simulink model "cav_pid"  (R2026b)
settings: Solver=ode4  StopTime=P.Tsim  FixedStep=P.dt
InitFcn:
  | P = cav_params(); road = make_road(P.road.segments, P.road.ds, P.road.transition); mpcverbosity off;
libraries: slpidlib x3, autolibshared x1
settings Model: Creator=za  LastModifiedBy=za
settings SolverCC: AutoInsertRateTranBlk=on

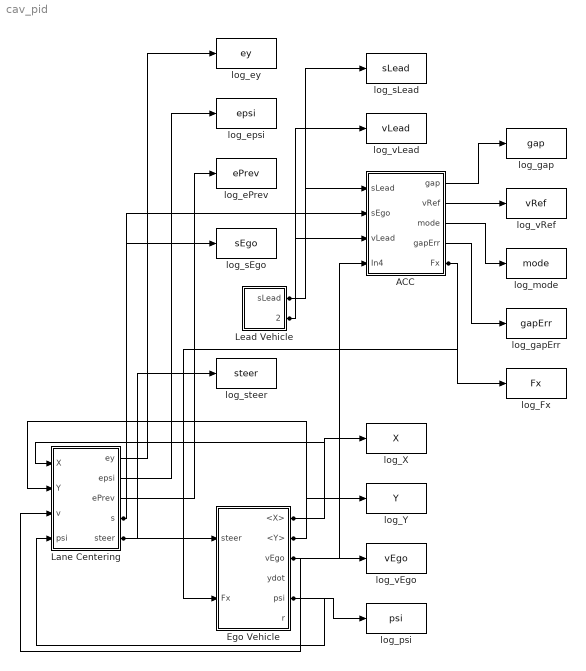
== system cav_pid ==
  ACC : Subsystem
  Ego Vehicle : Subsystem
  Lane Centering : Subsystem
  Lead Vehicle : Subsystem
  log_Fx : ToWorkspace  VariableName=Fx  SaveFormat=Timeseries  SampleTime=P.Ts
  log_X : ToWorkspace  VariableName=X  SaveFormat=Timeseries  SampleTime=P.Ts
  log_Y : ToWorkspace  VariableName=Y  SaveFormat=Timeseries  SampleTime=P.Ts
  log_ePrev : ToWorkspace  VariableName=ePrev  SaveFormat=Timeseries  SampleTime=P.Ts
  log_epsi : ToWorkspace  VariableName=epsi  SaveFormat=Timeseries  SampleTime=P.Ts
  log_ey : ToWorkspace  VariableName=ey  SaveFormat=Timeseries  SampleTime=P.Ts
  log_gap : ToWorkspace  VariableName=gap  SaveFormat=Timeseries  SampleTime=P.Ts
  log_gapErr : ToWorkspace  VariableName=gapErr  SaveFormat=Timeseries  SampleTime=P.Ts
  log_mode : ToWorkspace  VariableName=mode  SaveFormat=Timeseries  SampleTime=P.Ts
  log_psi : ToWorkspace  VariableName=psi  SaveFormat=Timeseries  SampleTime=P.Ts
  log_sEgo : ToWorkspace  VariableName=sEgo  SaveFormat=Timeseries  SampleTime=P.Ts
  log_sLead : ToWorkspace  VariableName=sLead  SaveFormat=Timeseries  SampleTime=P.Ts
  log_steer : ToWorkspace  VariableName=steer  SaveFormat=Timeseries  SampleTime=P.Ts
  log_vEgo : ToWorkspace  VariableName=vEgo  SaveFormat=Timeseries  SampleTime=P.Ts
  log_vLead : ToWorkspace  VariableName=vLead  SaveFormat=Timeseries  SampleTime=P.Ts
  log_vRef : ToWorkspace  VariableName=vRef  SaveFormat=Timeseries  SampleTime=P.Ts
  wires:
  ACC/4(gapErr) -> log_gapErr/1
  ACC/3(mode) -> log_mode/1
  ACC/5(Fx) -> log_Fx/1, Ego Vehicle/2(Fx)
  Lane Centering/5(steer) -> Ego Vehicle/1(steer), log_steer/1
  Lane Centering/1(ey) -> log_ey/1
  Lane Centering/2(epsi) -> log_epsi/1
  Ego Vehicle/2(<Y>) -> log_Y/1, Lane Centering/2(Y)
  Lane Centering/3(ePrev) -> log_ePrev/1
  Lead Vehicle/2(vLead) -> log_vLead/1, ACC/3(vLead)
  ACC/2(vRef) -> log_vRef/1
  Lane Centering/4(s) -> log_sEgo/1, ACC/2(sEgo)
  Lead Vehicle/1(sLead) -> ACC/1(sLead), log_sLead/1
  Ego Vehicle/5(psi) -> log_psi/1, Lane Centering/4(psi)
  Ego Vehicle/3(vEgo) -> log_vEgo/1, ACC/4(In4), Lane Centering/3(v)
  Ego Vehicle/1(<X>) -> log_X/1, Lane Centering/1(X)
  ACC/1(gap) -> log_gap/1

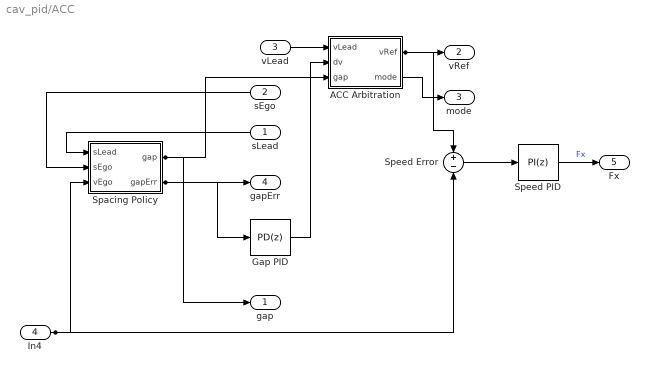
== system cav_pid/ACC ==
  sLead : Inport
  sEgo : Inport  Port=2
  vLead : Inport  Port=3
  In4 : Inport  Port=4
  ACC Arbitration : MATLAB Function  TreatAsAtomicUnit=on
  Gap PID : slpidlib/PID Controller  Controller=PD  Form=Parallel  TimeDomain=Discrete-time  UseExternalTs=off  SampleTime=P.Ts  IntegratorMethod=Forward Euler  FilterMethod=Backward Euler  ControllerParametersSource=internal  P=P.acc.gap.P  I=1  UseKiTs=off  D=P.acc.gap.D  UseExternalDerivativeSource=off  N=P.acc.gap.N  UseFilter=on  TunerSelectOption=Transfer Function Based (PID Tuner App)  InitialConditionSource=internal  InitialConditionForIntegrator=0  InitialConditionForFilter=0  DifferentiatorICPrevScaledInput=0  ExternalReset=none  TrackingMode=off  Kt=1  LimitOutput=on  SatLimitsSource=internal  UpperSaturationLimit=P.acc.gap.dvMax  LowerSaturationLimit=-P.acc.gap.dvMax  LinearizeAsGain=off  AntiWindupMode=none  Kb=1  LimitIntegrator=off  UpperIntegratorSaturationLimit=inf  LowerIntegratorSaturationLimit=-inf  POutMin=[]  POutMax=[]  IOutMin=[]  IOutMax=[]  DOutMin=[]  DOutMax=[]  NOutMin=[]  NOutMax=[]  SumOutMin=[]  SumOutMax=[]  SaturationOutMin=[]  SaturationOutMax=[]  PParamMin=[]  PParamMax=[]  IParamMin=[]  IParamMax=[]  DParamMin=[]  DParamMax=[]  NParamMin=[]  NParamMax=[]  KbParamMin=[]  KbParamMax=[]  KtParamMin=[]  KtParamMax=[]  KbOutMin=[]  KbOutMax=[]  KtOutMin=[]  KtOutMax=[]  IntegratorOutMin=[]  IntegratorOutMax=[]  FilterOutMin=[]  FilterOutMax=[]  SumI1OutMin=[]  SumI1OutMax=[]  SumI2OutMin=[]  SumI2OutMax=[]  SumI3OutMin=[]  SumI3OutMax=[]  SumI4OutMin=[]  SumI4OutMax=[]  SumDOutMin=[]  SumDOutMax=[]  DifferentiatorOutMin=[]  DifferentiatorOutMax=[]  FilterDiffOutCoefMin=[]  FilterDiffOutCoefMax=[]  ReciprocalOutMin=[]  ReciprocalOutMax=[]  SumDenOutMin=[]  SumDenOutMax=[]  SumNumOutMin=[]  SumNumOutMax=[]  DivideOutMin=[]  DivideOutMax=[]  UdiffTsProdOutMin=[]  UdiffTsProdOutMax=[]  NTsProdOutMin=[]  NTsProdOutMax=[]  UintegralTsProdOutMin=[]  UintegralTsProdOutMax=[]  UngainTsProdOutMin=[]  UngainTsProdOutMax=[]  ClampingZeroOutDataTypeStr=Inherit: Inherit via back propagation  ClampingZeroOutMin=[]  ClampingZeroOutMax=[]  FilterDenConstantOutDataTypeStr=Inherit: Inherit via back propagation  FilterDenConstantOutMin=[]  FilterDenConstantOutMax=[]  PCopyOutDataTypeStr=Inherit: Inherit via back propagation  PCopyOutMin=[]  PCopyOutMax=[]  NCopyOutDataTypeStr=Inherit: Inherit via back propagation  NCopyOutMin=[]  NCopyOutMax=[]  IntegratorContinuousStateAttributes=''  IntegratorStateMustResolveToSignalObject=off  IntegratorRTWStateStorageClass=Auto  FilterContinuousStateAttributes=''  FilterStateMustResolveToSignalObject=off  FilterRTWStateStorageClass=Auto  ParallelPVariant=InternalParameters  IdealPVariant=Disabled  IVariant=Disabled  DVariant=InternalParameters  IntegratorVariant=Disabled  SatVariant=Enabled  AWVariant=Disabled  PCopyVariant=Disabled  TRVariant=Disabled  FdbkBlocksVariant=Forward  IdealPFdbkVariant=Disabled  SatFdbkVariant=Disabled  DerivativeFilterVariant=BackwardEulerFilter  NVariant=InternalParameters  NCopyVariant=InternalParameters  FilterICVariant=InternalICsFilter  IntegratorICVariant=Disabled  ExternalResetVariant=Disabled  TRSumVariant=Passthrough  SumFdbkVariant=Disabled  SumVariant=Sum_PD  TsampFilterVariant=InternalTs  TsampNgainVariant=Passthrough  TsampIntegralVariant=Disabled_SignalSpec  ExternalSaturationOutDataTypeStr=Inherit: Same as second input  DerivativeSourceVariant=ErrorSignal  PreIntVariant=InternalPreInt
      settings: LibrarySourceBlock=simulink/Discrete/Discrete PID Controller
  Spacing Policy : MATLAB Function  TreatAsAtomicUnit=on
  Speed Error : Sum  Inputs=+-
  Speed PID : slpidlib/PID Controller  Controller=PI  Form=Parallel  TimeDomain=Discrete-time  UseExternalTs=off  SampleTime=P.Ts  IntegratorMethod=Forward Euler  FilterMethod=Forward Euler  ControllerParametersSource=internal  P=P.acc.speed.P  I=P.acc.speed.I  UseKiTs=off  D=0  UseExternalDerivativeSource=off  N=100  UseFilter=on  TunerSelectOption=Transfer Function Based (PID Tuner App)  InitialConditionSource=internal  InitialConditionForIntegrator=150  InitialConditionForFilter=0  DifferentiatorICPrevScaledInput=0  ExternalReset=none  TrackingMode=off  Kt=1  LimitOutput=on  SatLimitsSource=internal  UpperSaturationLimit=P.acc.FxMax  LowerSaturationLimit=P.acc.FxMin  LinearizeAsGain=off  AntiWindupMode=clamping  Kb=1  LimitIntegrator=off  UpperIntegratorSaturationLimit=inf  LowerIntegratorSaturationLimit=-inf  POutMin=[]  POutMax=[]  IOutMin=[]  IOutMax=[]  DOutMin=[]  DOutMax=[]  NOutMin=[]  NOutMax=[]  SumOutMin=[]  SumOutMax=[]  SaturationOutMin=[]  SaturationOutMax=[]  PParamMin=[]  PParamMax=[]  IParamMin=[]  IParamMax=[]  DParamMin=[]  DParamMax=[]  NParamMin=[]  NParamMax=[]  KbParamMin=[]  KbParamMax=[]  KtParamMin=[]  KtParamMax=[]  KbOutMin=[]  KbOutMax=[]  KtOutMin=[]  KtOutMax=[]  IntegratorOutMin=[]  IntegratorOutMax=[]  FilterOutMin=[]  FilterOutMax=[]  SumI1OutMin=[]  SumI1OutMax=[]  SumI2OutMin=[]  SumI2OutMax=[]  SumI3OutMin=[]  SumI3OutMax=[]  SumI4OutMin=[]  SumI4OutMax=[]  SumDOutMin=[]  SumDOutMax=[]  DifferentiatorOutMin=[]  DifferentiatorOutMax=[]  FilterDiffOutCoefMin=[]  FilterDiffOutCoefMax=[]  ReciprocalOutMin=[]  ReciprocalOutMax=[]  SumDenOutMin=[]  SumDenOutMax=[]  SumNumOutMin=[]  SumNumOutMax=[]  DivideOutMin=[]  DivideOutMax=[]  UdiffTsProdOutMin=[]  UdiffTsProdOutMax=[]  NTsProdOutMin=[]  NTsProdOutMax=[]  UintegralTsProdOutMin=[]  UintegralTsProdOutMax=[]  UngainTsProdOutMin=[]  UngainTsProdOutMax=[]  ClampingZeroOutDataTypeStr=Inherit: Inherit via back propagation  ClampingZeroOutMin=[]  ClampingZeroOutMax=[]  FilterDenConstantOutDataTypeStr=Inherit: Inherit via back propagation  FilterDenConstantOutMin=[]  FilterDenConstantOutMax=[]  PCopyOutDataTypeStr=Inherit: Inherit via back propagation  PCopyOutMin=[]  PCopyOutMax=[]  NCopyOutDataTypeStr=Inherit: Inherit via back propagation  NCopyOutMin=[]  NCopyOutMax=[]  IntegratorContinuousStateAttributes=''  IntegratorStateMustResolveToSignalObject=off  IntegratorRTWStateStorageClass=Auto  FilterContinuousStateAttributes=''  FilterStateMustResolveToSignalObject=off  FilterRTWStateStorageClass=Auto  ParallelPVariant=InternalParameters  IdealPVariant=Disabled  IVariant=InternalParameters  DVariant=Disabled  IntegratorVariant=Discrete  SatVariant=Enabled  AWVariant=DiscClampingParallel  PCopyVariant=Disabled  TRVariant=Disabled  FdbkBlocksVariant=Forward  IdealPFdbkVariant=Disabled  SatFdbkVariant=Disabled  DerivativeFilterVariant=Disabled  NVariant=Disabled  NCopyVariant=Disabled_SignalSpec  FilterICVariant=Disabled  IntegratorICVariant=InternalICs  ExternalResetVariant=Disabled  TRSumVariant=Passthrough  SumFdbkVariant=Disabled  SumVariant=Sum_PI  TsampFilterVariant=InternalTs  TsampNgainVariant=Passthrough  TsampIntegralVariant=Disabled_SignalSpec  ExternalSaturationOutDataTypeStr=Inherit: Same as second input  DerivativeSourceVariant=Disabled  PreIntVariant=InternalPreInt
      settings: LibrarySourceBlock=simulink/Discrete/Discrete PID Controller
  gap : Outport
  vRef : Outport  Port=2
  mode : Outport  Port=3
  gapErr : Outport  Port=4
  Fx : Outport  Port=5
  wires:
  Speed PID/1 -> Fx/1  "Fx"
  Speed Error/1 -> Speed PID/1
  ACC Arbitration/2(mode) -> mode/1
  ACC Arbitration/1(vRef) -> vRef/1, Speed Error/1
  Gap PID/1 -> ACC Arbitration/2(dv)
  sLead/1 -> Spacing Policy/1(sLead)
  sEgo/1 -> Spacing Policy/2(sEgo)
  Spacing Policy/2(gapErr) -> gapErr/1, Gap PID/1
  Spacing Policy/1(gap) -> gap/1, ACC Arbitration/3(gap)
  vLead/1 -> ACC Arbitration/1(vLead)
  In4/1 -> Spacing Policy/3(vEgo), Speed Error/2

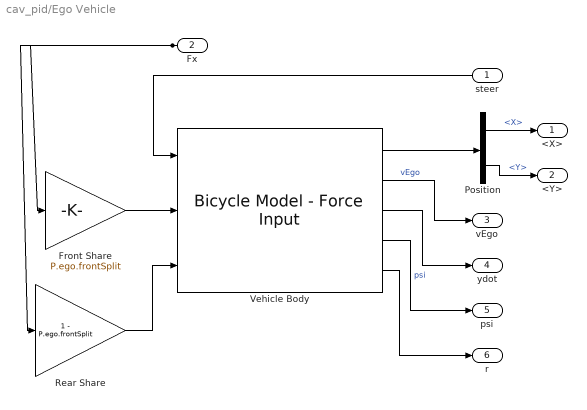
== system cav_pid/Ego Vehicle ==
  steer : Inport
  Fx : Inport  Port=2
  Front Share : Gain  Gain=P.ego.frontSplit
  Position : BusSelector  OutputSignals=InertFrm.Cg.Disp.X,InertFrm.Cg.Disp.Y
  Rear Share : Gain  Gain=1 - P.ego.frontSplit
  Vehicle Body : autolibshared/Bicycle Model - Force Input  trackMode=Single (bicycle)  inputMode=External longitudinal forces  frontSteerMode=on  rearSteerMode=off  windMode=off  muMode=off  extFMode=off  extMMode=off  aMode=2  NF=2  NR=2  m=P.ego.m  a=P.ego.a  b=P.ego.b  h=0.35  X_o=0  xdot_o=P.ego.v0  CalphaMode=Constant  sigmaMode=on  w=[1.4,1.4]  Cy_f=P.ego.Cyf  Cy_r=P.ego.Cyr  sigma_f=.1  sigma_r=.1  alpha_f_brk=[-.1 .1]  Cy_f_data=[-9e3 9e3]  alpha_r_brk=[-.1 .1]  Cy_r_data=[-9e3 9e3]  Y_o=0  ydot_o=0  Izz=P.ego.Izz  psi_o=0  r_o=0  Af=2  Cd=.3  Cl=.1  Cpm=.1  beta_w=[0,0.1745,0.3491,0.5236,0.6981,0.8727,1.0472,1.2217,1.3963,1.5708]  Cs=[0.1000,0.1000,0.1000,0.1000,0.1000,0.1000,0.1000,0.1000,0.1000,0.1000]  Cym=[0,0,0.0667,0.1000,0.1333,0.1667,0.2000,0.2333,0.2667,0.3000]  Pabs=101325  Tair=273  g=9.81  mu=1  xdot_tol=0.1  Fznom=5000  Fxtire_sat=1e6  Fytire_sat=1e6  longOff=0  latOff=0  vertOff=0.35
      settings: LibrarySourceBlock=vehdynlibeom/Bicycle Model - Force Input
  <X> : Outport
  <Y> : Outport  Port=2
  vEgo : Outport  Port=3
  ydot : Outport  Port=4
  psi : Outport  Port=5
  r : Outport  Port=6
  wires:
  Position/2 -> <Y>/1  "<Y>"
  Position/1 -> <X>/1  "<X>"
  steer/1 -> Vehicle Body/1
  Vehicle Body/5 -> r/1
  Vehicle Body/4 -> psi/1  "psi"
  Vehicle Body/3 -> ydot/1
  Vehicle Body/2 -> vEgo/1  "vEgo"
  Vehicle Body/1 -> Position/1
  Fx/1 -> Front Share/1, Rear Share/1
  Rear Share/1 -> Vehicle Body/3
  Front Share/1 -> Vehicle Body/2

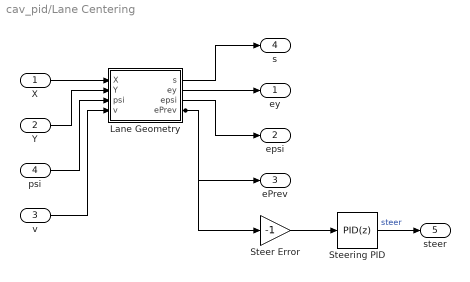
== system cav_pid/Lane Centering ==
  X : Inport
  Y : Inport  Port=2
  v : Inport  Port=3
  psi : Inport  Port=4
  Lane Geometry : MATLAB Function  TreatAsAtomicUnit=on
  Steer Error : Gain  Gain=-1
  Steering PID : slpidlib/PID Controller  Controller=PID  Form=Parallel  TimeDomain=Discrete-time  UseExternalTs=off  SampleTime=P.Ts  IntegratorMethod=Forward Euler  FilterMethod=Backward Euler  ControllerParametersSource=internal  P=P.lat.P  I=P.lat.I  UseKiTs=off  D=P.lat.D  UseExternalDerivativeSource=off  N=P.lat.N  UseFilter=on  TunerSelectOption=Transfer Function Based (PID Tuner App)  InitialConditionSource=internal  InitialConditionForIntegrator=0  InitialConditionForFilter=0  DifferentiatorICPrevScaledInput=0  ExternalReset=none  TrackingMode=off  Kt=1  LimitOutput=on  SatLimitsSource=internal  UpperSaturationLimit=P.lat.maxSteer  LowerSaturationLimit=-P.lat.maxSteer  LinearizeAsGain=off  AntiWindupMode=clamping  Kb=1  LimitIntegrator=off  UpperIntegratorSaturationLimit=inf  LowerIntegratorSaturationLimit=-inf  POutMin=[]  POutMax=[]  IOutMin=[]  IOutMax=[]  DOutMin=[]  DOutMax=[]  NOutMin=[]  NOutMax=[]  SumOutMin=[]  SumOutMax=[]  SaturationOutMin=[]  SaturationOutMax=[]  PParamMin=[]  PParamMax=[]  IParamMin=[]  IParamMax=[]  DParamMin=[]  DParamMax=[]  NParamMin=[]  NParamMax=[]  KbParamMin=[]  KbParamMax=[]  KtParamMin=[]  KtParamMax=[]  KbOutMin=[]  KbOutMax=[]  KtOutMin=[]  KtOutMax=[]  IntegratorOutMin=[]  IntegratorOutMax=[]  FilterOutMin=[]  FilterOutMax=[]  SumI1OutMin=[]  SumI1OutMax=[]  SumI2OutMin=[]  SumI2OutMax=[]  SumI3OutMin=[]  SumI3OutMax=[]  SumI4OutMin=[]  SumI4OutMax=[]  SumDOutMin=[]  SumDOutMax=[]  DifferentiatorOutMin=[]  DifferentiatorOutMax=[]  FilterDiffOutCoefMin=[]  FilterDiffOutCoefMax=[]  ReciprocalOutMin=[]  ReciprocalOutMax=[]  SumDenOutMin=[]  SumDenOutMax=[]  SumNumOutMin=[]  SumNumOutMax=[]  DivideOutMin=[]  DivideOutMax=[]  UdiffTsProdOutMin=[]  UdiffTsProdOutMax=[]  NTsProdOutMin=[]  NTsProdOutMax=[]  UintegralTsProdOutMin=[]  UintegralTsProdOutMax=[]  UngainTsProdOutMin=[]  UngainTsProdOutMax=[]  ClampingZeroOutDataTypeStr=Inherit: Inherit via back propagation  ClampingZeroOutMin=[]  ClampingZeroOutMax=[]  FilterDenConstantOutDataTypeStr=Inherit: Inherit via back propagation  FilterDenConstantOutMin=[]  FilterDenConstantOutMax=[]  PCopyOutDataTypeStr=Inherit: Inherit via back propagation  PCopyOutMin=[]  PCopyOutMax=[]  NCopyOutDataTypeStr=Inherit: Inherit via back propagation  NCopyOutMin=[]  NCopyOutMax=[]  IntegratorContinuousStateAttributes=''  IntegratorStateMustResolveToSignalObject=off  IntegratorRTWStateStorageClass=Auto  FilterContinuousStateAttributes=''  FilterStateMustResolveToSignalObject=off  FilterRTWStateStorageClass=Auto  ParallelPVariant=InternalParameters  IdealPVariant=Disabled  IVariant=InternalParameters  DVariant=InternalParameters  IntegratorVariant=Discrete  SatVariant=Enabled  AWVariant=DiscClampingParallel  PCopyVariant=Disabled  TRVariant=Disabled  FdbkBlocksVariant=Forward  IdealPFdbkVariant=Disabled  SatFdbkVariant=Disabled  DerivativeFilterVariant=BackwardEulerFilter  NVariant=InternalParameters  NCopyVariant=InternalParameters  FilterICVariant=InternalICsFilter  IntegratorICVariant=InternalICs  ExternalResetVariant=Disabled  TRSumVariant=Passthrough  SumFdbkVariant=Disabled  SumVariant=Sum_PID  TsampFilterVariant=InternalTs  TsampNgainVariant=Passthrough  TsampIntegralVariant=Disabled_SignalSpec  ExternalSaturationOutDataTypeStr=Inherit: Same as second input  DerivativeSourceVariant=ErrorSignal  PreIntVariant=InternalPreInt
      settings: LibrarySourceBlock=simulink/Discrete/Discrete PID Controller
  ey : Outport
  epsi : Outport  Port=2
  ePrev : Outport  Port=3
  s : Outport  Port=4
  steer : Outport  Port=5
  wires:
  Steering PID/1 -> steer/1  "steer"
  Steer Error/1 -> Steering PID/1
  Lane Geometry/4(ePrev) -> ePrev/1, Steer Error/1
  Lane Geometry/3(epsi) -> epsi/1
  Lane Geometry/2(ey) -> ey/1
  Lane Geometry/1(s) -> s/1
  v/1 -> Lane Geometry/4(v)
  psi/1 -> Lane Geometry/3(psi)
  Y/1 -> Lane Geometry/2(Y)
  X/1 -> Lane Geometry/1(X)

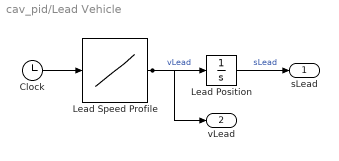
== system cav_pid/Lead Vehicle ==
  Clock : Clock
  Lead Position : Integrator  InitialCondition=P.lead.s0
  Lead Speed Profile : Lookup_n-D  NumberOfTableDimensions=1  BreakpointsForDimension1=P.lead.t  Table=P.lead.v  ExtrapMethod=Clip  InternalRulePriority=Speed  RndMeth=Simplest
  sLead : Outport
  vLead : Outport  Port=2
  wires:
  Lead Position/1 -> sLead/1  "sLead"
  Lead Speed Profile/1 -> Lead Position/1, vLead/1  "vLead"
  Clock/1 -> Lead Speed Profile/1

== matlab function cav_pid/ACC/Spacing Policy ==
  settings: updateMethod=DISCRETE  sampleTime=P.Ts
  data: sLead input; gap output; sEgo input; vEgo input; gapErr output; P parameter
function [gap, gapErr] = spacing_policy(sLead, sEgo, vEgo, P)
%Bumper-to-bumper gap and its error from the constant time-gap policy.
gap = sLead - sEgo - (P.ego.length + P.lead.length) / 2;
gapErr = gap - (P.acc.d0 + P.acc.Th * vEgo);
end

== matlab function cav_pid/Lane Centering/Lane Geometry ==
  settings: updateMethod=DISCRETE  sampleTime=P.Ts
  data: X input; s output; Y input; psi input; v input; ey output; epsi output; ePrev output; road parameter; P parameter
function [s, ey, epsi, ePrev] = lane_geometry(X, Y, psi, v, road, P)
%Arc length, lateral offset (left positive), heading error, and the
%lookahead error the steering PID drives to 0: the offset of a point L
%ahead along the heading, measured from the lane tangent at the car. It
%is zero only when the car is centered and aligned, so on a curve the
%integral term supplies the steady steering.
persistent idx
n = numel(road.x);
if isempty(idx)
    idx = nearest_index(road, X, Y, 1, n);
else
    idx = nearest_index(road, X, Y, max(1, idx - 40), min(n, idx + 200));
end
%Interpolate along the arc between centerline points, so heading and
%offset change smoothly instead of in steps of ds * curvature.
dx = X - road.x(idx);
dy = Y - road.y(idx);
along = cos(road.th(idx)) * dx + sin(road.th(idx)) * dy;
th = road.th(idx) + road.k(idx) * along;
ey = -sin(road.th(idx)) * dx + cos(road.th(idx)) * dy - road.k(idx) * along^2 / 2;
s = road.s(idx) + along;
epsi = atan2(sin(psi - th), cos(psi - th));
L = P.lat.L0 + P.lat.Tla * max(v, 0);
ePrev = ey + L * sin(epsi);
end

function best = nearest_index(road, X, Y, lo, hi)
best = lo;
bestD = inf;
for k = lo:hi
    d = (road.x(k) - X)^2 + (road.y(k) - Y)^2;
    if d < bestD
        bestD = d;
        best = k;
    end
end
end

== matlab function cav_pid/ACC/ACC Arbitration ==
  settings: updateMethod=DISCRETE  sampleTime=P.Ts
  data: vLead input; vRef output; dv input; gap input; mode output; P parameter
function [vRef, mode] = acc_arbitration(vLead, dv, gap, P)
%Speed command: the set speed, or the lead speed plus the gap correction,
%whichever is lower. mode is 1 for speed control and 2 for gap control.
vRef = P.acc.vSet;
mode = 1;
if gap < P.acc.range
    vGap = max(vLead + dv, 0);
    if vGap < vRef
        vRef = vGap;
        mode = 2;
    end
end
end
